simulink model "send_recv_cmd_sim"  (R2021a)
settings: Solver=FixedStepAuto  StartTime=0.0  StopTime=inf  FixedStep=0.002  RelTol=1e-3
settings Model: Creator=Ruixuan  LastModifiedBy=Ruixuan
settings SolverCC: ConcurrentTasks=on  PositivePriorityOrder=on
settings OptimizationCC: BlockReduction=off  DefaultParameterBehavior=Inlined  OptimizeBlockIOStorage=off
settings DebuggingCC: TasksWithSamePriorityMsg=none
settings HardwareCC: ProdBitPerLong=64  ProdLongLongMode=on  ProdHWDeviceType=Intel->x86-64 (Linux 64)
settings ModelReferenceCC: ModelReferenceNumInstancesAllowed=Single
settings RTWCC: Description=Simulink Real-Time  SystemTargetFile=slrealtime.tlc  TemplateMakefile=slrealtime_default_tmf  Toolchain=Simulink Real-Time Toolchain  BuildConfiguration=Faster Runs  CodeExecutionProfiling=on  TargetLang=C++

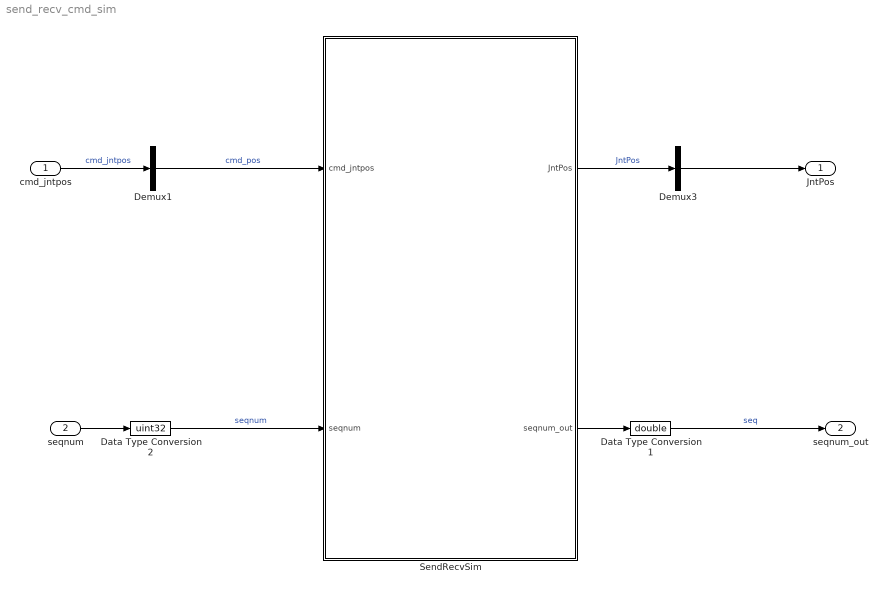
== system send_recv_cmd_sim ==
  cmd_jntpos : Inport
  seqnum : Inport  Port=2
  Data Type Conversion1 : DataTypeConversion  OutDataTypeStr=double
  Data Type Conversion2 : DataTypeConversion  OutDataTypeStr=uint32
  Demux1 : Demux  Outputs=[6]
  Demux3 : Demux  Outputs=[6]
  SendRecvSim : MATLAB Function  TreatAsAtomicUnit=on
  JntPos : Outport  VectorParamsAs1DForOutWhenUnconnected=off
  seqnum_out : Outport  Port=2  VectorParamsAs1DForOutWhenUnconnected=off
  wires:
  seqnum/1 -> Data Type Conversion2/1
  SendRecvSim/1(JntPos) -> Demux3/1  "JntPos"
  SendRecvSim/2(seqnum_out) -> Data Type Conversion1/1
  cmd_jntpos/1 -> Demux1/1  "cmd_jntpos"
  Data Type Conversion2/1 -> SendRecvSim/2(seqnum)  "seqnum"
  Demux1/1 -> SendRecvSim/1(cmd_jntpos)  "cmd_pos"
  Demux3/1 -> JntPos/1
  Data Type Conversion1/1 -> seqnum_out/1  "seq"

== matlab function send_recv_cmd_sim/SendRecvSim ==
  data: cmd_jntpos input; seqnum input; JntPos output; seqnum_out output
% This function simulates the robot feedback.
% Copyright (C) 2022  
% 
% Authors:
% Ruixuan Liu: ruixuanl@andrew.cmu.edu
% Rui Chen: ruic3@andrew.cmu.edu
% Changliu Liu : cliu6@andrew.cmu.edu
% 
% This program is free software; you can redistribute it and/or
% modify it under the terms of the GNU General Public License
% as published by the Free Software Foundation; either version 2
% of the License, or (at your option) any later version.
% 
% This program is distributed in the hope that it will be useful,
% but WITHOUT ANY WARRANTY; without even the implied warranty of
% MERCHANTABILITY or FITNESS FOR A PARTICULAR PURPOSE.  See the
% GNU General Public License for more details.
% 
% You should have received a copy of the GNU General Public License
% along with this program; if not, write to the Free Software
% Foundation, Inc., 51 Franklin Street, Fifth Floor, Boston, MA  02110-1301, USA.

function [JntPos, seqnum_out] = SendRecvSim(cmd_jntpos, seqnum)
    persistent m_jntpos;
    buff_size = 30;
    if isempty(m_jntpos)
        m_jntpos = zeros(6, buff_size);
    end
    m_jntpos(:, 1:buff_size-1) = m_jntpos(:, 2:buff_size);
    m_jntpos(:, buff_size) = cmd_jntpos(:);
    
    JntPos = m_jntpos(:, 1);

    seqnum_out = seqnum + uint32(1);
    if(seqnum_out > 100000000)
        seqnum_out = uint32(1);
    end
